simulink model "SystSansEtat"  (Simulink 10.1)
settings: Solver=ode8  StartTime=0.0  StopTime=100  RelTol=1e-3
libraries: simulink_extras x1
settings Model: Creator=iba  LastModifiedBy=iba
settings DataIOCC: LimitDataPoints=on  MaxDataPoints=10000  SaveFormat=Dataset  ReturnWorkspaceOutputs=on
settings OptimizationCC: DefaultParameterBehavior=Inlined  RollThreshold=2  LifeSpan=auto
settings DebuggingCC: AlgebraicLoopMsg=error  UnderspecifiedInitializationDetection=Simplified  MergeDetectMultiDrivingBlocksExec=error  SFUnexpectedBacktrackingDiag=error  SFNoUnconditionalDefaultTransitionDiag=error  SFExecutionAtInitializationDiag=warning  ArithmeticOperatorsInVariantConditions=error
settings HardwareCC: ProdBitPerPointer=64  ProdBitPerSizeT=64  ProdBitPerPtrDiffT=64  ProdLargestAtomicFloat=Float  ProdIntDivRoundTo=Zero  ProdEndianess=LittleEndian  ProdWordSize=64  ProdHWDeviceType=Intel->x86-64 (Windows64)
settings ModelReferenceCC: PropagateSignalLabelsOutOfModel=on
settings SFSimCC: SimUseLocalCustomCode=on  CustomCodeUndefinedFunction=FilterOut
settings RTWCC: RTWUseLocalCustomCode=on
settings CodeAppCC: StateflowObjectComments=off
settings GRTTargetCC: TargetLangStandard=C99 (ISO)  CombineOutputUpdateFcns=on  GRTInterface=off
settings ConfigComp: CovMetricSettings=dwe  CovHtmlReporting=off  CovSaveCumulativeToWorkspaceVar=off  CovSaveSingleToWorkspaceVar=off  CovExternalEMLEnable=on

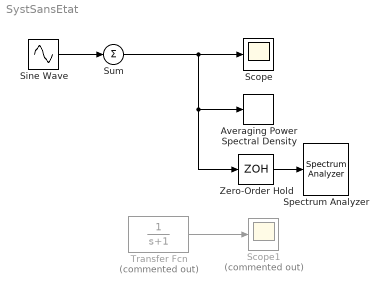
== system SystSansEtat ==
  Averaging Power Spectral Density : simulink_extras/Additional Sinks/Averaging Power Spectral Density  npts=128*4  fftpts=512*4  HowOften=64  sampleT=0.1
      settings: SourceProductBaseCode=SL
  Scope : Scope
  Scope1 : Scope  Commented=on
  Sine Wave : Sin  Amplitude=linspace(0.15,0.1,9)  Frequency=(1:0.5:5)  SampleTime=0
  Spectrum Analyzer : SpectrumAnalyzer
  Sum : Sum  Inputs=+
  Transfer Fcn : TransferFcn  Commented=on  Denominator=[1 1]
  Zero-Order Hold : ZeroOrderHold  SampleTime=0.1
  wires:
  Sine Wave/1 -> Sum/1
  Transfer Fcn/1 -> Scope1/1
  Sum/1 -> Scope/1, Zero-Order Hold/1, Averaging Power Spectral Density/1
  Zero-Order Hold/1 -> Spectrum Analyzer/1
